simulink model "auv_sonar_mission_controller"  (R2026a)
settings: Solver=FixedStepDiscrete  StopTime=t_mission_end  FixedStep=Ts_ping
PreLoadFcn:
  | % Self-healing path configuration for AUV Sonar Simulink Suite
  | m_file = get_param(bdroot, 'FileName');
  | if ~isempty(m_file)
  |     m_dir = fileparts(m_file);
  |     addpath(m_dir);
  |     addpath(fullfile(m_dir, '..'));
  | else
  |     if exist(fullfile(pwd, 'matlab', 'simulink'), 'dir')
  |         addpath(fullfile(pwd, 'matlab', 'simulink'));
  |         addpath(fullfile(pwd, 'matlab'));
  |     end
  | end
  | if exist('init_sonar_simulink', 'file') == 2
  |     init_sonar_simulink;
  | end
InitFcn:
  | % Self-healing path configuration for AUV Sonar Simulink Suite
  | m_file = get_param(bdroot, 'FileName');
  | if ~isempty(m_file)
  |     m_dir = fileparts(m_file);
  |     addpath(m_dir);
  |     addpath(fullfile(m_dir, '..'));
  | else
  |     if exist(fullfile(pwd, 'matlab', 'simulink'), 'dir')
  |         addpath(fullfile(pwd, 'matlab', 'simulink'));
  |         addpath(fullfile(pwd, 'matlab'));
  |     end
  | end
  | if exist('init_sonar_simulink', 'file') == 2
  |     init_sonar_simulink;
  | end
values from neighbouring files (symbols this model uses):
  Tp = 0.002    [sim_bridge_waveform.m]
undefined symbols (not defined in the file or in its folder): Ts_ping
settings Model: Creator=harsh  LastModifiedBy=harsh

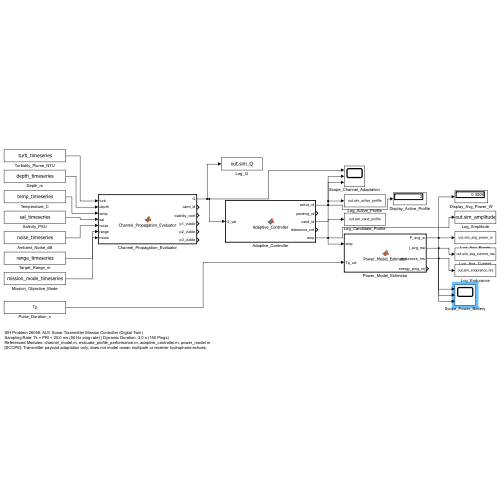
[thumbnail: Simulink's stored preview of the top-level diagram]
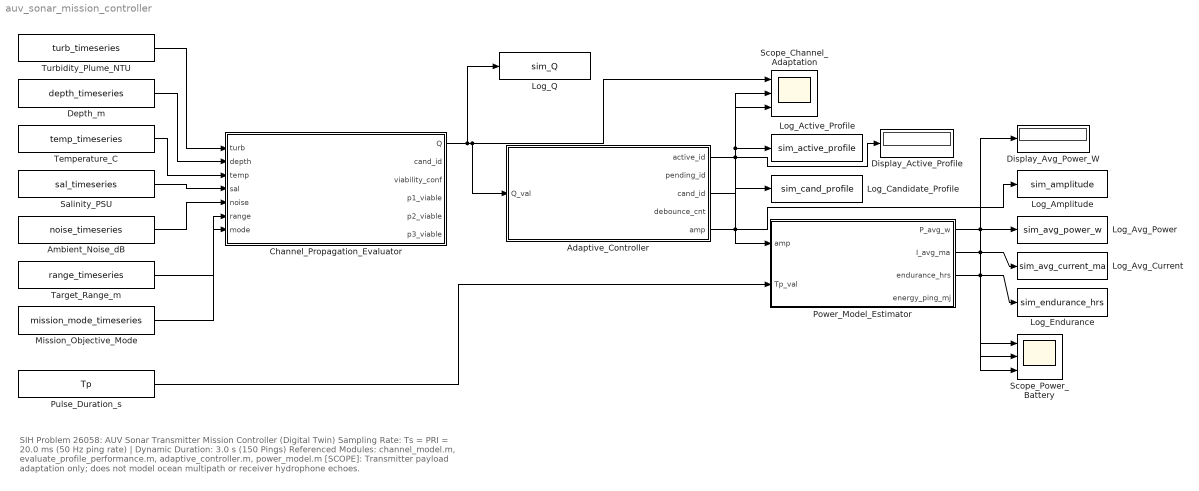
== system auv_sonar_mission_controller ==
  note: SIH Problem 26058: AUV Sonar Transmitter Mission Controller (Digital Twin)
      | Sampling Rate: Ts = PRI = 20.0 ms (50 Hz ping rate) | Dynamic Duration: 3.0 s (150 Pings)
      | Referenced Modules: channel_model.m, evaluate_profile_performance.m, adaptive_controller.m, power_model.m
      | [SCOPE]: Transmitter payload adaptation only; does not model ocean multipath or receiver hydrophone echoes.
  Adaptive_Controller : MATLAB Function  TreatAsAtomicUnit=on
  Ambient_Noise_dB : FromWorkspace  VariableName=noise_timeseries  SampleTime=Ts_ping  OutputAfterFinalValue=Holding final value
  Channel_Propagation_Evaluator : MATLAB Function  TreatAsAtomicUnit=on
  Depth_m : FromWorkspace  VariableName=depth_timeseries  SampleTime=Ts_ping  OutputAfterFinalValue=Holding final value
  Display_Active_Profile : Display
  Display_Avg_Power_W : Display
  Log_Active_Profile : ToWorkspace  VariableName=sim_active_profile  SampleTime=-1
  Log_Amplitude : ToWorkspace  VariableName=sim_amplitude  SampleTime=-1
  Log_Avg_Current : ToWorkspace  VariableName=sim_avg_current_ma  SampleTime=-1
  Log_Avg_Power : ToWorkspace  VariableName=sim_avg_power_w  SampleTime=-1
  Log_Candidate_Profile : ToWorkspace  VariableName=sim_cand_profile  SampleTime=-1
  Log_Endurance : ToWorkspace  VariableName=sim_endurance_hrs  SampleTime=-1
  Log_Q : ToWorkspace  VariableName=sim_Q  SampleTime=-1
  Mission_Objective_Mode : FromWorkspace  VariableName=mission_mode_timeseries  SampleTime=Ts_ping  OutputAfterFinalValue=Holding final value
  Power_Model_Estimator : MATLAB Function  TreatAsAtomicUnit=on
  Pulse_Duration_s : Constant  Value=Tp
  Salinity_PSU : FromWorkspace  VariableName=sal_timeseries  SampleTime=Ts_ping  OutputAfterFinalValue=Holding final value
  Scope_Channel_Adaptation : Scope  NumInputPorts=3
      settings: ActiveDisplayYMinimum=-0.76040750352451658  ActiveDisplayYMaximum=2.4211354652713917
  Scope_Power_Battery : Scope  NumInputPorts=3
      settings: ActiveDisplayYMinimum=-81.391538948690908  ActiveDisplayYMaximum=443.19454779875286
  Target_Range_m : FromWorkspace  VariableName=range_timeseries  SampleTime=Ts_ping  OutputAfterFinalValue=Holding final value
  Temperature_C : FromWorkspace  VariableName=temp_timeseries  SampleTime=Ts_ping  OutputAfterFinalValue=Holding final value
  Turbidity_Plume_NTU : FromWorkspace  VariableName=turb_timeseries  SampleTime=Ts_ping  OutputAfterFinalValue=Holding final value
  wires:
  Turbidity_Plume_NTU/1 -> Channel_Propagation_Evaluator/1(turb)
  Depth_m/1 -> Channel_Propagation_Evaluator/2(depth)
  Temperature_C/1 -> Channel_Propagation_Evaluator/3(temp)
  Salinity_PSU/1 -> Channel_Propagation_Evaluator/4(sal)
  Ambient_Noise_dB/1 -> Channel_Propagation_Evaluator/5(noise)
  Target_Range_m/1 -> Channel_Propagation_Evaluator/6(range)
  Mission_Objective_Mode/1 -> Channel_Propagation_Evaluator/7(mode)
  Channel_Propagation_Evaluator/1(Q) -> Adaptive_Controller/1(Q_val), Scope_Channel_Adaptation/1, Log_Q/1
  Adaptive_Controller/1(active_id) -> Log_Active_Profile/1, Scope_Channel_Adaptation/2, Display_Active_Profile/1
  Adaptive_Controller/3(cand_id) -> Log_Candidate_Profile/1
  Adaptive_Controller/5(amp) -> Power_Model_Estimator/1(amp), Log_Amplitude/1, Scope_Channel_Adaptation/3
  Pulse_Duration_s/1 -> Power_Model_Estimator/2(Tp_val)
  Power_Model_Estimator/1(P_avg_w) -> Log_Avg_Power/1, Display_Avg_Power_W/1, Scope_Power_Battery/1
  Power_Model_Estimator/2(I_avg_ma) -> Log_Avg_Current/1, Scope_Power_Battery/2
  Power_Model_Estimator/3(endurance_hrs) -> Log_Endurance/1, Scope_Power_Battery/3

== matlab function auv_sonar_mission_controller/Adaptive_Controller ==
  data: Q_val input; active_id output; pending_id output; cand_id output; debounce_cnt output; amp output
function [active_id, pending_id, cand_id, debounce_cnt, amp] = Adaptive_Controller(Q_val)
coder.extrinsic('sim_bridge_controller');
active_id = 2.0;
pending_id = 2.0;
cand_id = 2.0;
debounce_cnt = 0.0;
amp = 0.70;
[active_id, pending_id, cand_id, debounce_cnt, amp] = sim_bridge_controller(Q_val);
end

== matlab function auv_sonar_mission_controller/Channel_Propagation_Evaluator ==
  data: turb input; Q output; depth input; temp input; sal input; noise input; range input; mode input; cand_id output; viability_conf output; p1_viable output; p2_viable output; p3_viable output
function [Q, cand_id, viability_conf, p1_viable, p2_viable, p3_viable] = ...
    Channel_Propagation_Evaluator(turb, depth, temp, sal, noise, range, mode)
coder.extrinsic('sim_bridge_channel');
Q = 0.0;
cand_id = 1.0;
viability_conf = 0.0;
p1_viable = 0.0;
p2_viable = 0.0;
p3_viable = 0.0;
[Q, cand_id, viability_conf, p1_viable, p2_viable, p3_viable] = ...
    sim_bridge_channel(turb, depth, temp, sal, noise, range, mode);
end

== matlab function auv_sonar_mission_controller/Power_Model_Estimator ==
  data: amp input; P_avg_w output; Tp_val input; I_avg_ma output; endurance_hrs output; energy_ping_mj output
function [P_avg_w, I_avg_ma, endurance_hrs, energy_ping_mj] = Power_Model_Estimator(amp, Tp_val)
coder.extrinsic('sim_bridge_power');
P_avg_w = 0.0;
I_avg_ma = 0.0;
endurance_hrs = 0.0;
energy_ping_mj = 0.0;
[P_avg_w, I_avg_ma, endurance_hrs, energy_ping_mj] = sim_bridge_power(amp, Tp_val);
end
